simulink model "gap_generation_single_veh_state_machine"  (R2019a)
settings: Solver=VariableStepAuto  StartTime=0.0  StopTime=40  FixedStep=0.1  RelTol=1e-3
undefined symbols (not defined in the file): DiscIntNeverNeededParam
libraries: simulink x43, powerlib_meascontrol x5, autolibshared x5
(part 1 of 3)
settings Model: Creator=fvall  LastModifiedBy=fvall

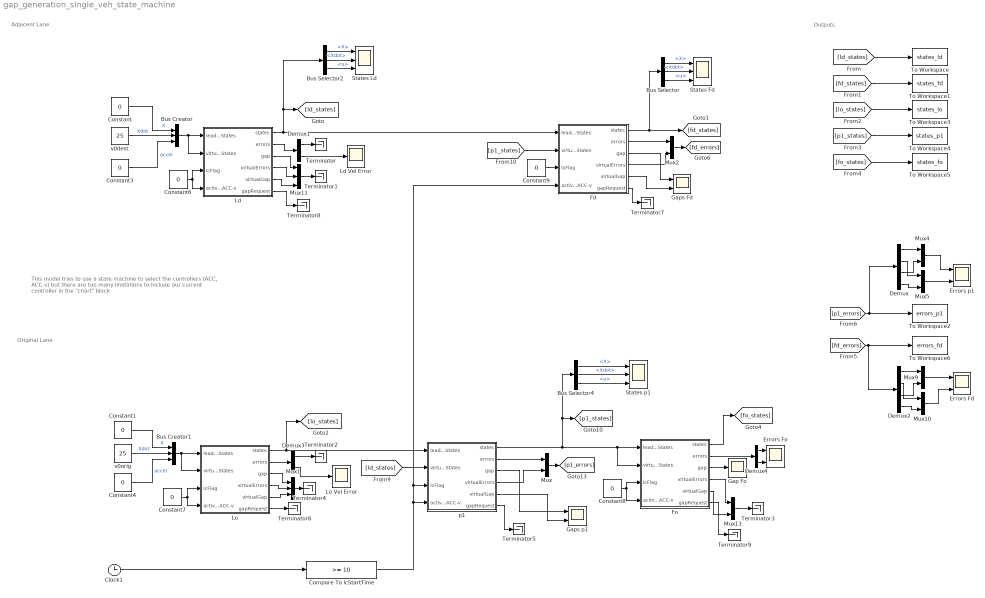
== system gap_generation_single_veh_state_machine ==
  note: Original Lane
  note: Adjacent Lane
  note: Outputs
  note: This model tries to use a state machine to select the controllers (ACC, ACC-v) but there are too many limitations to include our current controller in the "chart" block
  Bus Creator : BusCreator  Inputs=3
  Bus Creator1 : BusCreator  Inputs=3
  Bus Selector : BusSelector  OutputSignals=X,Xdot,u
  Bus Selector2 : BusSelector  OutputSignals=X,Xdot,u
  Bus Selector4 : BusSelector  OutputSignals=X,Xdot,u
  Clock1 : Clock
  Compare To lcStartTime : simulink/Logic and Bit Operations/Compare To Constant  relop=>=  const=10  OutDataTypeStr=boolean
  Constant{,1,3..4,6..9} (8 alike) : Constant  Value=0
  Demux : Demux
  Demux1 : Demux  Outputs=2
  Demux2 : Demux
  Demux3 : Demux  Outputs=2
  Demux4 : Demux  Outputs=2
  Errors Fd : Scope  NumInputPorts=2
  Errors Fo : Scope  NumInputPorts=2
  Errors p1 : Scope  NumInputPorts=2
  Fd : Subsystem  mask{m=2000, lf=2.5, lr=2.5, maxAcceleration=4, minAcceleration=-8, maxJerk=50, minJerk=-50, x0=20.2504, vx0=25, y0=3.6, h=0.63, d0=0.5004, minHeadwayError=-100, maxHeadwayError=3, velFilterGain=10, Kd=1.5652, Kp=2.2775, Ki=0.75, velKi=0.5, velKp=1.5, hFilterGain=0.5, vMin=18, l1=-2, maxComfAccel=2, minComfAccel=-2, maxComfJerk=10, minComfJerk=-10, hLc=2.215, d0Lc=0.5004}
      mask prompts: m "autoblks_shared:autoblkVehBody3DofLat:blkPrm_m"; lf "autoblks_shared:autoblkVehBody3DofLat:blkPrm_a"; lr "autoblks_shared:autoblkVehBody3DofLat:blkPrm_b"; maxAcceleration "Max Acceleration"; minAcceleration "Min Acceleration"; maxJerk "Max Jerk"; minJerk "Min Jerk"; x0 "autoblks_shared:autoblkVehBody3DofLat:blkPrm_X_o"; vx0 "autoblks_shared:autoblkVehBody3DofLat:blkPrm_xdot_o"; y0 "autoblks_shared:autoblkVehBody3DofLat:blkPrm_Y_o"; h "Time Headway"; d0 "Standstill Gap"; minHeadwayError "Min Headway Error"; maxHeadwayError "Max Headway Error"; velFilterGain "Velocity Filter Gain"; hFilterGain "Headway filter Gain"; vMin "Min Gap Gen Speed"; l1 "ACC-v Headway Error Threshold"; maxComfAccel "Max Comf Accel"; minComfAccel "Min Comf Accel"; maxComfJerk "Max Comf Jerk"; minComfJerk "Min Comf Jerk"; hLc "Time Headway LC"; d0Lc "Standstill Gap LC"
      mask TypeOptions m: Vehicle Body 3DOF Single Track/m
      mask TypeOptions lf: Vehicle Body 3DOF Single Track/a
      mask TypeOptions lr: Vehicle Body 3DOF Single Track/b
      mask TypeOptions x0: Vehicle Body 3DOF Single Track/X_o
      mask TypeOptions vx0: Vehicle Body 3DOF Single Track/xdot_o
      mask TypeOptions y0: Vehicle Body 3DOF Single Track/Y_o
      mask TypeOptions h: ACC/Headway error/h/Value
      mask TypeOptions d0: ACC/Headway error/d0/Value
      mask TypeOptions Kd: ACC/Kd/Gain
      mask TypeOptions Kp: ACC/Kp/Gain
      mask TypeOptions Ki: ACC/Ki/Gain
      mask TypeOptions velKi: ACC/velKi/Gain
      mask TypeOptions velKp: ACC/velKp/Gain
      mask TypeOptions hFilterGain: ACC/Headway error/hFilterGain/Gain
      mask TypeOptions vMin: ACC-v/vMin/Value
      mask TypeOptions l1:
      | ACC-v/Compare
      | To Constant/const
      mask TypeOptions hLc: ACC/Headway error/hLc/Value
      mask TypeOptions d0Lc: ACC/Headway error/d0Lc/Value
      mask DialogControl DescGroupVar Prompt: 3DOF Vehicle with ACC
      mask DialogControl DescTextVar Prompt: Vehicle with ACC. The vehicle model is Simulink's 3DOF single track vehicle body. The controller is a PID with constant headway including headway error saturation and filtered leader velocity.
      mask DialogControl VehParams Prompt: Vehicle Parameters
      mask DialogControl m Prompt: Vehicle mass, m [kg]:
      mask DialogControl lf Prompt: Longitudinal distance from center of mass to front axle, a [m]:
      mask DialogControl lr Prompt: Longitudinal distance from center of mass to rear axle, b [m]:
      mask DialogControl InitStates Prompt: Initial State
      mask DialogControl x0 Prompt: Initial inertial frame longitudinal position, X_o [m]:
      mask DialogControl vx0 Prompt: Initial longitudinal velocity, xdot_o [m/s]:
      mask DialogControl y0 Prompt: Initial inertial frame lateral displacement, Y_o [m]:
      mask DialogControl Container3 Prompt: Veh Following Parameters
      mask DialogControl VirtualFollParams Prompt: Virtual Veh Following Parameters
      mask DialogControl LCParams Prompt: Lane Change Params
  Fo : Subsystem  mask{m=2000, lf=2.5, lr=2.5, maxAcceleration=4, minAcceleration=-8, maxJerk=50, minJerk=-50, x0=0, vx0=25, y0=0, h=0.63, d0=0.5004, minHeadwayError=-100, maxHeadwayError=3, velFilterGain=10, Kd=1.5652, Kp=2.2775, Ki=0.75, velKi=0.5, velKp=1.5, hFilterGain=0.5, vMin=18, l1=-2, maxComfAccel=2, minComfAccel=-2, maxComfJerk=10, minComfJerk=-10, hLc=2.215, d0Lc=0.5004}
      mask prompts: m "autoblks_shared:autoblkVehBody3DofLat:blkPrm_m"; lf "autoblks_shared:autoblkVehBody3DofLat:blkPrm_a"; lr "autoblks_shared:autoblkVehBody3DofLat:blkPrm_b"; maxAcceleration "Max Acceleration"; minAcceleration "Min Acceleration"; maxJerk "Max Jerk"; minJerk "Min Jerk"; x0 "autoblks_shared:autoblkVehBody3DofLat:blkPrm_X_o"; vx0 "autoblks_shared:autoblkVehBody3DofLat:blkPrm_xdot_o"; y0 "autoblks_shared:autoblkVehBody3DofLat:blkPrm_Y_o"; h "Time Headway"; d0 "Standstill Gap"; minHeadwayError "Min Headway Error"; maxHeadwayError "Max Headway Error"; velFilterGain "Velocity Filter Gain"; hFilterGain "Headway filter Gain"; vMin "Min Gap Gen Speed"; l1 "ACC-v Headway Error Threshold"; maxComfAccel "Max Comf Accel"; minComfAccel "Min Comf Accel"; maxComfJerk "Max Comf Jerk"; minComfJerk "Min Comf Jerk"; hLc "Time Headway LC"; d0Lc "Standstill Gap LC"
      mask TypeOptions m: Vehicle Body 3DOF Single Track/m
      mask TypeOptions lf: Vehicle Body 3DOF Single Track/a
      mask TypeOptions lr: Vehicle Body 3DOF Single Track/b
      mask TypeOptions x0: Vehicle Body 3DOF Single Track/X_o
      mask TypeOptions vx0: Vehicle Body 3DOF Single Track/xdot_o
      mask TypeOptions y0: Vehicle Body 3DOF Single Track/Y_o
      mask TypeOptions h: ACC/Headway error/h/Value
      mask TypeOptions d0: ACC/Headway error/d0/Value
      mask TypeOptions Kd: ACC/Kd/Gain
      mask TypeOptions Kp: ACC/Kp/Gain
      mask TypeOptions Ki: ACC/Ki/Gain
      mask TypeOptions velKi: ACC/velKi/Gain
      mask TypeOptions velKp: ACC/velKp/Gain
      mask TypeOptions hFilterGain: ACC/Headway error/hFilterGain/Gain
      mask TypeOptions vMin: ACC-v/vMin/Value
      mask TypeOptions l1:
      | ACC-v/Compare
      | To Constant/const
      mask TypeOptions hLc: ACC/Headway error/hLc/Value
      mask TypeOptions d0Lc: ACC/Headway error/d0Lc/Value
      mask DialogControl DescGroupVar Prompt: 3DOF Vehicle with ACC
      mask DialogControl DescTextVar Prompt: Vehicle with ACC. The vehicle model is Simulink's 3DOF single track vehicle body. The controller is a PID with constant headway including headway error saturation and filtered leader velocity.
      mask DialogControl VehParams Prompt: Vehicle Parameters
      mask DialogControl m Prompt: Vehicle mass, m [kg]:
      mask DialogControl lf Prompt: Longitudinal distance from center of mass to front axle, a [m]:
      mask DialogControl lr Prompt: Longitudinal distance from center of mass to rear axle, b [m]:
      mask DialogControl InitStates Prompt: Initial State
      mask DialogControl x0 Prompt: Initial inertial frame longitudinal position, X_o [m]:
      mask DialogControl vx0 Prompt: Initial longitudinal velocity, xdot_o [m/s]:
      mask DialogControl y0 Prompt: Initial inertial frame lateral displacement, Y_o [m]:
      mask DialogControl Container3 Prompt: Veh Following Parameters
      mask DialogControl VirtualFollParams Prompt: Virtual Veh Following Parameters
      mask DialogControl LCParams Prompt: Lane Change Params
  Gap Fo : Scope
  Gaps Fd : Scope  NumInputPorts=2
  Gaps p1 : Scope  NumInputPorts=2
  Ld : Subsystem  mask{m=2000, lf=2.5, lr=2.5, maxAcceleration=4, minAcceleration=-8, maxJerk=50, minJerk=-50, x0=41.5008, vx0=25, y0=3.6, h=0.63, d0=0.5004, minHeadwayError=-100, maxHeadwayError=3, velFilterGain=10, Kd=1.5652, Kp=2.2775, Ki=0.75, velKi=0.5, velKp=1.5, hFilterGain=0.5, vMin=18, l1=-2, maxComfAccel=2, minComfAccel=-2, maxComfJerk=10, minComfJerk=-10, hLc=1.9025, d0Lc=0.5004}
      mask prompts: m "autoblks_shared:autoblkVehBody3DofLat:blkPrm_m"; lf "autoblks_shared:autoblkVehBody3DofLat:blkPrm_a"; lr "autoblks_shared:autoblkVehBody3DofLat:blkPrm_b"; maxAcceleration "Max Acceleration"; minAcceleration "Min Acceleration"; maxJerk "Max Jerk"; minJerk "Min Jerk"; x0 "autoblks_shared:autoblkVehBody3DofLat:blkPrm_X_o"; vx0 "autoblks_shared:autoblkVehBody3DofLat:blkPrm_xdot_o"; y0 "autoblks_shared:autoblkVehBody3DofLat:blkPrm_Y_o"; h "Time Headway"; d0 "Standstill Gap"; minHeadwayError "Min Headway Error"; maxHeadwayError "Max Headway Error"; velFilterGain "Velocity Filter Gain"; hFilterGain "Headway filter Gain"; vMin "Min Gap Gen Speed"; l1 "ACC-v Headway Error Threshold"; maxComfAccel "Max Comf Accel"; minComfAccel "Min Comf Accel"; maxComfJerk "Max Comf Jerk"; minComfJerk "Min Comf Jerk"; hLc "Time Headway LC"; d0Lc "Standstill Gap LC"
      mask TypeOptions m: Vehicle Body 3DOF Single Track/m
      mask TypeOptions lf: Vehicle Body 3DOF Single Track/a
      mask TypeOptions lr: Vehicle Body 3DOF Single Track/b
      mask TypeOptions x0: Vehicle Body 3DOF Single Track/X_o
      mask TypeOptions vx0: Vehicle Body 3DOF Single Track/xdot_o
      mask TypeOptions y0: Vehicle Body 3DOF Single Track/Y_o
      mask TypeOptions h: ACC/Headway error/h/Value
      mask TypeOptions d0: ACC/Headway error/d0/Value
      mask TypeOptions Kd: ACC/Kd/Gain
      mask TypeOptions Kp: ACC/Kp/Gain
      mask TypeOptions Ki: ACC/Ki/Gain
      mask TypeOptions velKi: ACC/velKi/Gain
      mask TypeOptions velKp: ACC/velKp/Gain
      mask TypeOptions hFilterGain: ACC/Headway error/hFilterGain/Gain
      mask TypeOptions vMin: ACC-v/vMin/Value
      mask TypeOptions l1:
      | ACC-v/Compare
      | To Constant/const
      mask TypeOptions hLc: ACC/Headway error/hLc/Value
      mask TypeOptions d0Lc: ACC/Headway error/d0Lc/Value
      mask DialogControl DescGroupVar Prompt: 3DOF Vehicle with ACC
      mask DialogControl DescTextVar Prompt: Vehicle with ACC. The vehicle model is Simulink's 3DOF single track vehicle body. The controller is a PID with constant headway including headway error saturation and filtered leader velocity.
      mask DialogControl VehParams Prompt: Vehicle Parameters
      mask DialogControl m Prompt: Vehicle mass, m [kg]:
      mask DialogControl lf Prompt: Longitudinal distance from center of mass to front axle, a [m]:
      mask DialogControl lr Prompt: Longitudinal distance from center of mass to rear axle, b [m]:
      mask DialogControl InitStates Prompt: Initial State
      mask DialogControl x0 Prompt: Initial inertial frame longitudinal position, X_o [m]:
      mask DialogControl vx0 Prompt: Initial longitudinal velocity, xdot_o [m/s]:
      mask DialogControl y0 Prompt: Initial inertial frame lateral displacement, Y_o [m]:
      mask DialogControl Container3 Prompt: Veh Following Parameters
      mask DialogControl VirtualFollParams Prompt: Virtual Veh Following Parameters
      mask DialogControl LCParams Prompt: Lane Change Params
  Ld Vel Error : Scope
  Lo : Subsystem  mask{m=2000, lf=2.5, lr=2.5, maxAcceleration=4, minAcceleration=-8, maxJerk=50, minJerk=-50, x0=42.5008, vx0=25, y0=0, h=0.63, d0=0.5004, minHeadwayError=-100, maxHeadwayError=3, velFilterGain=10, Kd=1.5652, Kp=2.2775, Ki=0.75, velKi=0.5, velKp=1.5, hFilterGain=0.5, vMin=18, l1=-2, maxComfAccel=2, minComfAccel=-2, maxComfJerk=10, minComfJerk=-10, hLc=1.9025, d0Lc=0.5004}
      mask prompts: m "autoblks_shared:autoblkVehBody3DofLat:blkPrm_m"; lf "autoblks_shared:autoblkVehBody3DofLat:blkPrm_a"; lr "autoblks_shared:autoblkVehBody3DofLat:blkPrm_b"; maxAcceleration "Max Acceleration"; minAcceleration "Min Acceleration"; maxJerk "Max Jerk"; minJerk "Min Jerk"; x0 "autoblks_shared:autoblkVehBody3DofLat:blkPrm_X_o"; vx0 "autoblks_shared:autoblkVehBody3DofLat:blkPrm_xdot_o"; y0 "autoblks_shared:autoblkVehBody3DofLat:blkPrm_Y_o"; h "Time Headway"; d0 "Standstill Gap"; minHeadwayError "Min Headway Error"; maxHeadwayError "Max Headway Error"; velFilterGain "Velocity Filter Gain"; hFilterGain "Headway filter Gain"; vMin "Min Gap Gen Speed"; l1 "ACC-v Headway Error Threshold"; maxComfAccel "Max Comf Accel"; minComfAccel "Min Comf Accel"; maxComfJerk "Max Comf Jerk"; minComfJerk "Min Comf Jerk"; hLc "Time Headway LC"; d0Lc "Standstill Gap LC"
      mask TypeOptions m: Vehicle Body 3DOF Single Track/m
      mask TypeOptions lf: Vehicle Body 3DOF Single Track/a
      mask TypeOptions lr: Vehicle Body 3DOF Single Track/b
      mask TypeOptions x0: Vehicle Body 3DOF Single Track/X_o
      mask TypeOptions vx0: Vehicle Body 3DOF Single Track/xdot_o
      mask TypeOptions y0: Vehicle Body 3DOF Single Track/Y_o
      mask TypeOptions h: ACC/Headway error/h/Value
      mask TypeOptions d0: ACC/Headway error/d0/Value
      mask TypeOptions Kd: ACC/Kd/Gain
      mask TypeOptions Kp: ACC/Kp/Gain
      mask TypeOptions Ki: ACC/Ki/Gain
      mask TypeOptions velKi: ACC/velKi/Gain
      mask TypeOptions velKp: ACC/velKp/Gain
      mask TypeOptions hFilterGain: ACC/Headway error/hFilterGain/Gain
      mask TypeOptions vMin: ACC-v/vMin/Value
      mask TypeOptions l1:
      | ACC-v/Compare
      | To Constant/const
      mask TypeOptions hLc: ACC/Headway error/hLc/Value
      mask TypeOptions d0Lc: ACC/Headway error/d0Lc/Value
      mask DialogControl DescGroupVar Prompt: 3DOF Vehicle with ACC
      mask DialogControl DescTextVar Prompt: Vehicle with ACC. The vehicle model is Simulink's 3DOF single track vehicle body. The controller is a PID with constant headway including headway error saturation and filtered leader velocity.
      mask DialogControl VehParams Prompt: Vehicle Parameters
      mask DialogControl m Prompt: Vehicle mass, m [kg]:
      mask DialogControl lf Prompt: Longitudinal distance from center of mass to front axle, a [m]:
      mask DialogControl lr Prompt: Longitudinal distance from center of mass to rear axle, b [m]:
      mask DialogControl InitStates Prompt: Initial State
      mask DialogControl x0 Prompt: Initial inertial frame longitudinal position, X_o [m]:
      mask DialogControl vx0 Prompt: Initial longitudinal velocity, xdot_o [m/s]:
      mask DialogControl y0 Prompt: Initial inertial frame lateral displacement, Y_o [m]:
      mask DialogControl Container3 Prompt: Veh Following Parameters
      mask DialogControl VirtualFollParams Prompt: Virtual Veh Following Parameters
      mask DialogControl LCParams Prompt: Lane Change Params
  Lo Vel Error : Scope
  Mux{,2,4..5,9..10,13} (7 alike) : Mux  Inputs=2
  Mux1 : Mux  Inputs=3
  Mux11 : Mux  Inputs=3
  States Fd : Scope  NumInputPorts=3
  States Ld : Scope  NumInputPorts=3
  States p1 : Scope  NumInputPorts=3
  Terminator{,1..9} (10 alike) : Terminator
  To Workspace : ToWorkspace  VariableName=states_ld  SampleTime=-1
  To Workspace1 : ToWorkspace  VariableName=states_fd  SampleTime=-1
  To Workspace2 : ToWorkspace  VariableName=errors_p1  SampleTime=-1
  To Workspace3 : ToWorkspace  VariableName=states_lo  SampleTime=-1
  To Workspace4 : ToWorkspace  VariableName=states_p1  SampleTime=-1
  To Workspace5 : ToWorkspace  VariableName=states_fo  SampleTime=-1
  To Workspace6 : ToWorkspace  VariableName=errors_fd  SampleTime=-1
  p1 : Subsystem  mask{m=2000, lf=2.5, lr=2.5, maxAcceleration=4, minAcceleration=-8, maxJerk=50, minJerk=-50, x0=21.2504, vx0=25, y0=0, h=0.63, d0=0.5004, minHeadwayError=-100, maxHeadwayError=3, velFilterGain=10, Kd=1.5652, Kp=2.2775, Ki=0.75, velKi=0.5, velKp=1.5, hFilterGain=0.5, vMin=18, l1=-2, maxComfAccel=2, minComfAccel=-2, maxComfJerk=10, minComfJerk=-10, hLc=2.215, d0Lc=0.5004}
      mask prompts: m "autoblks_shared:autoblkVehBody3DofLat:blkPrm_m"; lf "autoblks_shared:autoblkVehBody3DofLat:blkPrm_a"; lr "autoblks_shared:autoblkVehBody3DofLat:blkPrm_b"; maxAcceleration "Max Acceleration"; minAcceleration "Min Acceleration"; maxJerk "Max Jerk"; minJerk "Min Jerk"; x0 "autoblks_shared:autoblkVehBody3DofLat:blkPrm_X_o"; vx0 "autoblks_shared:autoblkVehBody3DofLat:blkPrm_xdot_o"; y0 "autoblks_shared:autoblkVehBody3DofLat:blkPrm_Y_o"; h "Time Headway"; d0 "Standstill Gap"; minHeadwayError "Min Headway Error"; maxHeadwayError "Max Headway Error"; velFilterGain "Velocity Filter Gain"; hFilterGain "Headway filter Gain"; vMin "Min Gap Gen Speed"; l1 "ACC-v Headway Error Threshold"; maxComfAccel "Max Comf Accel"; minComfAccel "Min Comf Accel"; maxComfJerk "Max Comf Jerk"; minComfJerk "Min Comf Jerk"; hLc "Time Headway LC"; d0Lc "Standstill Gap LC"
      mask TypeOptions m: Vehicle Body 3DOF Single Track/m
      mask TypeOptions lf: Vehicle Body 3DOF Single Track/a
      mask TypeOptions lr: Vehicle Body 3DOF Single Track/b
      mask TypeOptions x0: Vehicle Body 3DOF Single Track/X_o
      mask TypeOptions vx0: Vehicle Body 3DOF Single Track/xdot_o
      mask TypeOptions y0: Vehicle Body 3DOF Single Track/Y_o
      mask TypeOptions h: ACC/Headway error/h/Value
      mask TypeOptions d0: ACC/Headway error/d0/Value
      mask TypeOptions Kd: ACC/Kd/Gain
      mask TypeOptions Kp: ACC/Kp/Gain
      mask TypeOptions Ki: ACC/Ki/Gain
      mask TypeOptions velKi: ACC/velKi/Gain
      mask TypeOptions velKp: ACC/velKp/Gain
      mask TypeOptions hFilterGain: ACC/Headway error/hFilterGain/Gain
      mask TypeOptions vMin: ACC-v/vMin/Value
      mask TypeOptions l1:
      | ACC-v/Compare
      | To Constant/const
      mask TypeOptions hLc: ACC/Headway error/hLc/Value
      mask TypeOptions d0Lc: ACC/Headway error/d0Lc/Value
      mask DialogControl DescGroupVar Prompt: 3DOF Vehicle with ACC
      mask DialogControl DescTextVar Prompt: Vehicle with ACC. The vehicle model is Simulink's 3DOF single track vehicle body. The controller is a PID with constant headway including headway error saturation and filtered leader velocity.
      mask DialogControl VehParams Prompt: Vehicle Parameters
      mask DialogControl m Prompt: Vehicle mass, m [kg]:
      mask DialogControl lf Prompt: Longitudinal distance from center of mass to front axle, a [m]:
      mask DialogControl lr Prompt: Longitudinal distance from center of mass to rear axle, b [m]:
      mask DialogControl InitStates Prompt: Initial State
      mask DialogControl x0 Prompt: Initial inertial frame longitudinal position, X_o [m]:
      mask DialogControl vx0 Prompt: Initial longitudinal velocity, xdot_o [m/s]:
      mask DialogControl y0 Prompt: Initial inertial frame lateral displacement, Y_o [m]:
      mask DialogControl Container3 Prompt: Veh Following Parameters
      mask DialogControl VirtualFollParams Prompt: Virtual Veh Following Parameters
      mask DialogControl LCParams Prompt: Lane Change Params
  v0dest : Constant  Value=25
  v0orig : Constant  Value=25
  wires:
  Clock1/1 -> Compare To lcStartTime/1
  Lo/1(states) -> p1/1(leaderStates), [lo_states]
  Bus Selector4/3 -> States p1/3  "<u>"
  Bus Selector4/2 -> States p1/2  "<Xdot>"
  Bus Selector4/1 -> States p1/1  "<X>"
  p1/2(errors) -> Mux/1
  Ld/2(errors) -> Demux1/1
  Bus Selector2/3 -> States Ld/3  "<u>"
  Fd/6(gapRequest) -> Terminator7/1
  Fd/4(virtualErrors) -> Mux2/2
  Fd/5(virtualGap) -> Gaps Fd/2
  Fd/1(states) -> Bus Selector/1, [fd_states]
  Ld/3(gap) -> Mux11/1
  Fd/3(gap) -> Gaps Fd/1
  Mux11/1 -> Terminator1/1
  Fd/2(errors) -> Mux2/1
  Demux1/2 -> Ld Vel Error/1
  Bus Selector2/2 -> States Ld/2  "<Xdot>"
  Bus Selector2/1 -> States Ld/1  "<X>"
  Ld/6(gapRequest) -> Terminator8/1
  Bus Selector/1 -> States Fd/1  "<X>"
  [p1_states] -> Fd/2(virtualLeaderStates)
  Constant9/1 -> Fd/3(lcFlag)
  Ld/5(virtualGap) -> Mux11/3
  Bus Selector/3 -> States Fd/3  "<u>"
  Constant6/1 -> Ld/4(activate ACC-v), Ld/3(lcFlag)
  Ld/4(virtualErrors) -> Mux11/2
  Bus Selector/2 -> States Fd/2  "<Xdot>"
  Ld/1(states) -> Fd/1(leaderStates), Bus Selector2/1, [ld_states]
  v0dest/1 -> Bus Creator/2  "Xdot"
  Constant3/1 -> Bus Creator/3  "accel"
  Mux2/1 -> [fd_errors]
  Constant/1 -> Bus Creator/1  "X"
  Demux1/1 -> Terminator/1
  Bus Creator/1 -> Ld/1(leaderStates), Ld/2(virtualLeaderStates)
  Lo/2(errors) -> Demux3/1
  Demux3/1 -> Terminator2/1
  Bus Creator1/1 -> Lo/1(leaderStates), Lo/2(virtualLeaderStates)
  Constant7/1 -> Lo/3(lcFlag), Lo/4(activate ACC-v)
  v0orig/1 -> Bus Creator1/2  "Xdot"
  Constant4/1 -> Bus Creator1/3  "accel"
  Constant1/1 -> Bus Creator1/1  "X"
  Demux3/2 -> Lo Vel Error/1
  Mux13/1 -> Terminator3/1
  Fo/2(errors) -> Demux4/1
  Fo/4(virtualErrors) -> Mux13/1
  Fo/3(gap) -> Gap Fo/1
  Demux4/2 -> Errors Fo/2
  Constant8/1 -> Fo/4(activate ACC-v), Fo/3(lcFlag)
  Demux4/1 -> Errors Fo/1
  Fo/1(states) -> [fo_states]
  p1/1(states) -> Fo/2(virtualLeaderStates), Fo/1(leaderStates), Bus Selector4/1, [p1_states]
  Fo/5(virtualGap) -> Mux13/2
  [ld_states] -> p1/2(virtualLeaderStates)
  Compare To lcStartTime/1 -> Fd/4(activate ACC-v), p1/3(lcFlag), p1/4(activate ACC-v)
  p1/3(gap) -> Gaps p1/1
  [fd_states] -> To Workspace1/1
  [lo_states] -> To Workspace3/1
  Mux10/1 -> Errors Fd/2
  Mux4/1 -> Errors p1/1
  Demux/2 -> Mux5/1
  Mux9/1 -> Errors Fd/1
  Demux/3 -> Mux4/2
  Demux/1 -> Mux4/1
  Mux5/1 -> Errors p1/2
  Demux2/2 -> Mux10/1
  Demux2/3 -> Mux9/2
  [p1_errors] -> To Workspace2/1, Demux/1
  [fd_errors] -> Demux2/1, To Workspace6/1
  [p1_states] -> To Workspace4/1
  Demux2/4 -> Mux10/2
  [ld_states] -> To Workspace/1
  Demux/4 -> Mux5/2
  [fo_states] -> To Workspace5/1
  Demux2/1 -> Mux9/1
  Mux/1 -> [p1_errors]
  p1/4(virtualErrors) -> Mux/2
  p1/5(virtualGap) -> Gaps p1/2
  p1/6(gapRequest) -> Terminator5/1
  Lo/3(gap) -> Mux1/1
  Lo/4(virtualErrors) -> Mux1/2
  Lo/5(virtualGap) -> Mux1/3
  Mux1/1 -> Terminator4/1
  Lo/6(gapRequest) -> Terminator6/1
  Fo/6(gapRequest) -> Terminator9/1

== system gap_generation_single_veh_state_machine/Fd ==
  leaderStates : Inport
  virtualLeaderStates : Inport  Port=2
  lcFlag : Inport  Port=3
  activate ACC-v : Inport  Port=4
  ACC : Subsystem
  ACC-v : Subsystem
  AND : Logic  Inputs=3  IconShape=distinctive  AllPortsSameDT=off  OutDataTypeStr=boolean
  Abs : Abs
  Abs1 : Abs  ZeroCross=off
  Bus Creator : BusCreator  Inputs=4
  Bus Selector : BusSelector  OutputSignals=InertFrm.RearAxl.Disp.X,InertFrm.RearAxl.Disp.Y,InertFrm.RearAxl.Vel.Xdot
  Compare To Constant : simulink/Logic and Bit Operations/Compare To Constant  relop=<=  const=0.5  OutDataTypeStr=boolean
  Compare To Constant1 : simulink/Logic and Bit Operations/Compare To Constant  relop=<=  const=0.5  OutDataTypeStr=boolean
  Constant : Constant  Value=0
  Constant1 : Constant  Value=maxAcceleration+1
  Gain : Gain  Gain=m/2
  Min : MinMax  Inputs=2
  Mux1 : Mux  Inputs=6
  On Delay : powerlib_meascontrol/Logic/On Delay  DelayType=On delay  delay=1  ic=0  Ts=0
      settings: SourceProductName=Simscape Electrical
  Scope : Scope  NumInputPorts=2
  Scope1 : Scope  NumInputPorts=3
  Signal Specification : SignalSpecification  Dimensions=1
  Switch : Switch  Criteria=u2 > Threshold
  Terminator : Terminator
  Transport Delay : TransportDelay
  Triggered Subsystem : Subsystem  TreatAsAtomicUnit=on
  Vehicle Body 3DOF Single Track : autolibshared/Vehicle Body 3DOF Single Track  trackMode=Single (bicycle)  inputMode=External longitudinal forces  frontSteerMode=on  rearSteerMode=off  windMode=off  muMode=off  extFMode=off  extMMode=off  extXo=off  extpsio=off  extxdoto=off  extro=off  extYo=off  extTamb=off  extydoto=off  aMode=2  NF=2  NR=2  m=m  a=lf  b=lr  h=0.35  X_o=x0  xdot_o=vx0  CalphaMode=off  sigmaMode=on  d=0  w=[1.4,1.4]  Cy_f=12e3  Cy_r=11e3  sigma_f=.1  sigma_r=.1  alpha_f_brk=[-.1 .1]  Cy_f_data=[-9e3 9e3]  alpha_r_brk=[-.1 .1]  Cy_r_data=[-9e3 9e3]  Y_o=y0  ydot_o=0  Izz=4000  psi_o=0  r_o=0  Af=2  Cd=.3  Cl=.1  Cpm=.1  beta_w=[0:0.01:0.3]  Cs=[0:0.03:0.9]  Cym=[0:0.01:0.3]  Pabs=101325  Tair=273  g=9.81  mu=1  xdot_tol=.01  Fznom=5000  Fxtire_sat=7e4  Fytire_sat=7e4  longOff=0  latOff=0  vertOff=0  wrapAng=off
      settings: SourceProductName=Powertrain Blockset  SourceProductBaseCode=PW
  states : Outport
  errors : Outport  Port=2
  gap : Outport  Port=3
  virtualErrors : Outport  Port=4
  virtualGap : Outport  Port=5
  gapRequest : Outport  Port=6
  wires:
  Abs1/1 -> Compare To Constant1/1
  Abs/1 -> Compare To Constant/1
  Transport Delay/1 -> Abs/1
  Compare To Constant/1 -> AND/2
  Triggered Subsystem/1(Out1) -> Scope/2, gapRequest/1
  On Delay/1 -> Triggered Subsystem/1(In1), AND/3
  Compare To Constant1/1 -> AND/1, Scope/1
  AND/1 -> Triggered Subsystem/Trigger
  Constant1/1 -> Switch/3
  activate ACC-v/1 -> Switch/2, ACC-v/3(activate)
  Signal Specification/1 -> Gain/1, Bus Creator/4, Abs1/1, Transport Delay/1
  Bus Selector/2 -> Bus Creator/2  "<Y>"
  ACC-v/3(gap) -> virtualGap/1
  ACC-v/2(errors) -> virtualErrors/1
  ACC-v/1(u) -> Switch/1
  Switch/1 -> Min/2, Scope1/2  "acc-v"
  lcFlag/1 -> ACC/3(lcFlag), On Delay/1, ACC-v/4(lcFlag)
  ACC/2(errors) -> errors/1
  virtualLeaderStates/1 -> ACC-v/2(leaderStates)
  leaderStates/1 -> ACC/2(leaderStates)
  Bus Creator/1 -> states/1, ACC-v/1(currentStates), ACC/1(currentStates)
  ACC/3(gap) -> gap/1
  Mux1/1 -> Terminator/1
  Vehicle Body 3DOF Single Track/7 -> Mux1/6
  Vehicle Body 3DOF Single Track/6 -> Mux1/5
  Vehicle Body 3DOF Single Track/5 -> Mux1/4
  Vehicle Body 3DOF Single Track/2 -> Mux1/1
  Vehicle Body 3DOF Single Track/3 -> Mux1/2
  Vehicle Body 3DOF Single Track/4 -> Mux1/3
  Vehicle Body 3DOF Single Track/1 -> Bus Selector/1
  Constant/1 -> Vehicle Body 3DOF Single Track/1
  Gain/1 -> Vehicle Body 3DOF Single Track/2, Vehicle Body 3DOF Single Track/3
  ACC/1(u) -> Min/1, Scope1/1  "acc"
  Min/1 -> Signal Specification/1, Scope1/3  "u"
  Bus Selector/1 -> Bus Creator/1  "<X>"
  Bus Selector/3 -> Bus Creator/3  "<Xdot>"

== system gap_generation_single_veh_state_machine/Fo ==
  leaderStates : Inport
  virtualLeaderStates : Inport  Port=2
  lcFlag : Inport  Port=3
  activate ACC-v : Inport  Port=4
  ACC : Subsystem
  ACC-v : Subsystem
  AND : Logic  Inputs=3  IconShape=distinctive  AllPortsSameDT=off  OutDataTypeStr=boolean
  Abs : Abs
  Abs1 : Abs  ZeroCross=off
  Bus Creator : BusCreator  Inputs=4
  Bus Selector : BusSelector  OutputSignals=InertFrm.RearAxl.Disp.X,InertFrm.RearAxl.Disp.Y,InertFrm.RearAxl.Vel.Xdot
  Compare To Constant : simulink/Logic and Bit Operations/Compare To Constant  relop=<=  const=0.5  OutDataTypeStr=boolean
  Compare To Constant1 : simulink/Logic and Bit Operations/Compare To Constant  relop=<=  const=0.5  OutDataTypeStr=boolean
  Constant : Constant  Value=0
  Constant1 : Constant  Value=maxAcceleration+1
  Gain : Gain  Gain=m/2
  Min : MinMax  Inputs=2
  Mux1 : Mux  Inputs=6
  On Delay : powerlib_meascontrol/Logic/On Delay  DelayType=On delay  delay=1  ic=0  Ts=0
      settings: SourceProductName=Simscape Electrical
  Scope : Scope  NumInputPorts=2
  Scope1 : Scope  NumInputPorts=3
  Signal Specification : SignalSpecification  Dimensions=1
  Switch : Switch  Criteria=u2 > Threshold
  Terminator : Terminator
  Transport Delay : TransportDelay
  Triggered Subsystem : Subsystem  TreatAsAtomicUnit=on
  Vehicle Body 3DOF Single Track : autolibshared/Vehicle Body 3DOF Single Track  trackMode=Single (bicycle)  inputMode=External longitudinal forces  frontSteerMode=on  rearSteerMode=off  windMode=off  muMode=off  extFMode=off  extMMode=off  extXo=off  extpsio=off  extxdoto=off  extro=off  extYo=off  extTamb=off  extydoto=off  aMode=2  NF=2  NR=2  m=m  a=lf  b=lr  h=0.35  X_o=x0  xdot_o=vx0  CalphaMode=off  sigmaMode=on  d=0  w=[1.4,1.4]  Cy_f=12e3  Cy_r=11e3  sigma_f=.1  sigma_r=.1  alpha_f_brk=[-.1 .1]  Cy_f_data=[-9e3 9e3]  alpha_r_brk=[-.1 .1]  Cy_r_data=[-9e3 9e3]  Y_o=y0  ydot_o=0  Izz=4000  psi_o=0  r_o=0  Af=2  Cd=.3  Cl=.1  Cpm=.1  beta_w=[0:0.01:0.3]  Cs=[0:0.03:0.9]  Cym=[0:0.01:0.3]  Pabs=101325  Tair=273  g=9.81  mu=1  xdot_tol=.01  Fznom=5000  Fxtire_sat=7e4  Fytire_sat=7e4  longOff=0  latOff=0  vertOff=0  wrapAng=off
      settings: SourceProductName=Powertrain Blockset  SourceProductBaseCode=PW
  states : Outport
  errors : Outport  Port=2
  gap : Outport  Port=3
  virtualErrors : Outport  Port=4
  virtualGap : Outport  Port=5
  gapRequest : Outport  Port=6
  wires:
  Abs1/1 -> Compare To Constant1/1
  Abs/1 -> Compare To Constant/1
  Transport Delay/1 -> Abs/1
  Compare To Constant/1 -> AND/2
  Triggered Subsystem/1(Out1) -> Scope/2, gapRequest/1
  On Delay/1 -> Triggered Subsystem/1(In1), AND/3
  Compare To Constant1/1 -> AND/1, Scope/1
  AND/1 -> Triggered Subsystem/Trigger
  Constant1/1 -> Switch/3
  activate ACC-v/1 -> Switch/2, ACC-v/3(activate)
  Signal Specification/1 -> Gain/1, Bus Creator/4, Abs1/1, Transport Delay/1
  Bus Selector/2 -> Bus Creator/2  "<Y>"
  ACC-v/3(gap) -> virtualGap/1
  ACC-v/2(errors) -> virtualErrors/1
  ACC-v/1(u) -> Switch/1
  Switch/1 -> Min/2, Scope1/2  "acc-v"
  lcFlag/1 -> ACC/3(lcFlag), On Delay/1, ACC-v/4(lcFlag)
  ACC/2(errors) -> errors/1
  virtualLeaderStates/1 -> ACC-v/2(leaderStates)
  leaderStates/1 -> ACC/2(leaderStates)
  Bus Creator/1 -> states/1, ACC-v/1(currentStates), ACC/1(currentStates)
  ACC/3(gap) -> gap/1
  Mux1/1 -> Terminator/1
  Vehicle Body 3DOF Single Track/7 -> Mux1/6
  Vehicle Body 3DOF Single Track/6 -> Mux1/5
  Vehicle Body 3DOF Single Track/5 -> Mux1/4
  Vehicle Body 3DOF Single Track/2 -> Mux1/1
  Vehicle Body 3DOF Single Track/3 -> Mux1/2
  Vehicle Body 3DOF Single Track/4 -> Mux1/3
  Vehicle Body 3DOF Single Track/1 -> Bus Selector/1
  Constant/1 -> Vehicle Body 3DOF Single Track/1
  Gain/1 -> Vehicle Body 3DOF Single Track/2, Vehicle Body 3DOF Single Track/3
  ACC/1(u) -> Min/1, Scope1/1  "acc"
  Min/1 -> Signal Specification/1, Scope1/3  "u"
  Bus Selector/1 -> Bus Creator/1  "<X>"
  Bus Selector/3 -> Bus Creator/3  "<Xdot>"

== system gap_generation_single_veh_state_machine/Ld ==
  leaderStates : Inport
  virtualLeaderStates : Inport  Port=2
  lcFlag : Inport  Port=3
  activate ACC-v : Inport  Port=4
  ACC : Subsystem
  ACC-v : Subsystem
  AND : Logic  Inputs=3  IconShape=distinctive  AllPortsSameDT=off  OutDataTypeStr=boolean
  Abs : Abs
  Abs1 : Abs  ZeroCross=off
  Bus Creator : BusCreator  Inputs=4  OutDataTypeStr=Bus: vehStates
  Bus Selector : BusSelector  OutputSignals=InertFrm.RearAxl.Disp.X,InertFrm.RearAxl.Disp.Y,InertFrm.RearAxl.Vel.Xdot
  Compare To Constant : simulink/Logic and Bit Operations/Compare To Constant  relop=<=  const=0.5  OutDataTypeStr=boolean
  Compare To Constant1 : simulink/Logic and Bit Operations/Compare To Constant  relop=<=  const=0.5  OutDataTypeStr=boolean
  Constant : Constant  Value=0
  Constant1 : Constant  Value=maxAcceleration+1
  Gain : Gain  Gain=m/2
  Min : MinMax  Inputs=2
  Mux1 : Mux  Inputs=6
  On Delay : powerlib_meascontrol/Logic/On Delay  DelayType=On delay  delay=1  ic=0  Ts=0
      settings: SourceProductName=Simscape Electrical
  Scope : Scope  NumInputPorts=2
  Scope1 : Scope  NumInputPorts=3
  Signal Specification : SignalSpecification  Dimensions=1
  Switch : Switch  Criteria=u2 > Threshold
  Terminator : Terminator
  Transport Delay : TransportDelay
  Triggered Subsystem : Subsystem  TreatAsAtomicUnit=on
  Vehicle Body 3DOF Single Track : autolibshared/Vehicle Body 3DOF Single Track  trackMode=Single (bicycle)  inputMode=External longitudinal forces  frontSteerMode=on  rearSteerMode=off  windMode=off  muMode=off  extFMode=off  extMMode=off  extXo=off  extpsio=off  extxdoto=off  extro=off  extYo=off  extTamb=off  extydoto=off  aMode=2  NF=2  NR=2  m=m  a=lf  b=lr  h=0.35  X_o=x0  xdot_o=vx0  CalphaMode=off  sigmaMode=on  d=0  w=[1.4,1.4]  Cy_f=12e3  Cy_r=11e3  sigma_f=.1  sigma_r=.1  alpha_f_brk=[-.1 .1]  Cy_f_data=[-9e3 9e3]  alpha_r_brk=[-.1 .1]  Cy_r_data=[-9e3 9e3]  Y_o=y0  ydot_o=0  Izz=4000  psi_o=0  r_o=0  Af=2  Cd=.3  Cl=.1  Cpm=.1  beta_w=[0:0.01:0.3]  Cs=[0:0.03:0.9]  Cym=[0:0.01:0.3]  Pabs=101325  Tair=273  g=9.81  mu=1  xdot_tol=.01  Fznom=5000  Fxtire_sat=7e4  Fytire_sat=7e4  longOff=0  latOff=0  vertOff=0  wrapAng=off
      settings: SourceProductName=Powertrain Blockset  SourceProductBaseCode=PW
  states : Outport
  errors : Outport  Port=2
  gap : Outport  Port=3
  virtualErrors : Outport  Port=4
  virtualGap : Outport  Port=5
  gapRequest : Outport  Port=6
  wires:
  Bus Selector/3 -> Bus Creator/3  "<Xdot>"
  Bus Selector/1 -> Bus Creator/1  "<X>"
  Min/1 -> Scope1/3, Signal Specification/1  "u"
  ACC/1(u) -> Scope1/1, Min/1  "acc"
  Gain/1 -> Vehicle Body 3DOF Single Track/3, Vehicle Body 3DOF Single Track/2
  Constant/1 -> Vehicle Body 3DOF Single Track/1
  Vehicle Body 3DOF Single Track/1 -> Bus Selector/1
  Vehicle Body 3DOF Single Track/4 -> Mux1/3
  Vehicle Body 3DOF Single Track/3 -> Mux1/2
  Vehicle Body 3DOF Single Track/2 -> Mux1/1
  Vehicle Body 3DOF Single Track/5 -> Mux1/4
  Vehicle Body 3DOF Single Track/6 -> Mux1/5
  Vehicle Body 3DOF Single Track/7 -> Mux1/6
  Mux1/1 -> Terminator/1
  ACC/3(gap) -> gap/1
  Bus Creator/1 -> ACC/1(currentStates), ACC-v/1(currentStates), states/1
  leaderStates/1 -> ACC/2(leaderStates)
  virtualLeaderStates/1 -> ACC-v/2(leaderStates)
  ACC/2(errors) -> errors/1
  lcFlag/1 -> ACC-v/4(lcFlag), On Delay/1, ACC/3(lcFlag)
  Switch/1 -> Scope1/2, Min/2  "acc-v"
  ACC-v/1(u) -> Switch/1
  ACC-v/2(errors) -> virtualErrors/1
  ACC-v/3(gap) -> virtualGap/1
  Bus Selector/2 -> Bus Creator/2  "<Y>"
  Signal Specification/1 -> Transport Delay/1, Abs1/1, Bus Creator/4, Gain/1
  activate ACC-v/1 -> ACC-v/3(activate), Switch/2
  Constant1/1 -> Switch/3
  AND/1 -> Triggered Subsystem/Trigger
  Compare To Constant1/1 -> Scope/1, AND/1
  On Delay/1 -> AND/3, Triggered Subsystem/1(In1)
  Triggered Subsystem/1(Out1) -> gapRequest/1, Scope/2
  Compare To Constant/1 -> AND/2
  Transport Delay/1 -> Abs/1
  Abs/1 -> Compare To Constant/1
  Abs1/1 -> Compare To Constant1/1

== system gap_generation_single_veh_state_machine/Lo ==
  leaderStates : Inport
  virtualLeaderStates : Inport  Port=2
  lcFlag : Inport  Port=3
  activate ACC-v : Inport  Port=4
  ACC : Subsystem
  ACC-v : Subsystem
  AND : Logic  Inputs=3  IconShape=distinctive  AllPortsSameDT=off  OutDataTypeStr=boolean
  Abs : Abs
  Abs1 : Abs  ZeroCross=off
  Bus Creator : BusCreator  Inputs=4  OutDataTypeStr=Bus: vehStates
  Bus Selector : BusSelector  OutputSignals=InertFrm.RearAxl.Disp.X,InertFrm.RearAxl.Disp.Y,InertFrm.RearAxl.Vel.Xdot
  Compare To Constant : simulink/Logic and Bit Operations/Compare To Constant  relop=<=  const=0.5  OutDataTypeStr=boolean
  Compare To Constant1 : simulink/Logic and Bit Operations/Compare To Constant  relop=<=  const=0.5  OutDataTypeStr=boolean
  Constant : Constant  Value=0
  Constant1 : Constant  Value=maxAcceleration+1
  Gain : Gain  Gain=m/2
  Min : MinMax  Inputs=2
  Mux1 : Mux  Inputs=6
  On Delay : powerlib_meascontrol/Logic/On Delay  DelayType=On delay  delay=1  ic=0  Ts=0
      settings: SourceProductName=Simscape Electrical
  Scope : Scope  NumInputPorts=2
  Scope1 : Scope  NumInputPorts=3
  Signal Specification : SignalSpecification  Dimensions=1
  Switch : Switch  Criteria=u2 > Threshold
  Terminator : Terminator
  Transport Delay : TransportDelay
  Triggered Subsystem : Subsystem  TreatAsAtomicUnit=on
  Vehicle Body 3DOF Single Track : autolibshared/Vehicle Body 3DOF Single Track  trackMode=Single (bicycle)  inputMode=External longitudinal forces  frontSteerMode=on  rearSteerMode=off  windMode=off  muMode=off  extFMode=off  extMMode=off  extXo=off  extpsio=off  extxdoto=off  extro=off  extYo=off  extTamb=off  extydoto=off  aMode=2  NF=2  NR=2  m=m  a=lf  b=lr  h=0.35  X_o=x0  xdot_o=vx0  CalphaMode=off  sigmaMode=on  d=0  w=[1.4,1.4]  Cy_f=12e3  Cy_r=11e3  sigma_f=.1  sigma_r=.1  alpha_f_brk=[-.1 .1]  Cy_f_data=[-9e3 9e3]  alpha_r_brk=[-.1 .1]  Cy_r_data=[-9e3 9e3]  Y_o=y0  ydot_o=0  Izz=4000  psi_o=0  r_o=0  Af=2  Cd=.3  Cl=.1  Cpm=.1  beta_w=[0:0.01:0.3]  Cs=[0:0.03:0.9]  Cym=[0:0.01:0.3]  Pabs=101325  Tair=273  g=9.81  mu=1  xdot_tol=.01  Fznom=5000  Fxtire_sat=7e4  Fytire_sat=7e4  longOff=0  latOff=0  vertOff=0  wrapAng=off
      settings: SourceProductName=Powertrain Blockset  SourceProductBaseCode=PW
  states : Outport
  errors : Outport  Port=2
  gap : Outport  Port=3
  virtualErrors : Outport  Port=4
  virtualGap : Outport  Port=5
  gapRequest : Outport  Port=6
  wires:
  Abs1/1 -> Compare To Constant1/1
  Abs/1 -> Compare To Constant/1
  Transport Delay/1 -> Abs/1
  Compare To Constant/1 -> AND/2
  Triggered Subsystem/1(Out1) -> Scope/2, gapRequest/1
  On Delay/1 -> Triggered Subsystem/1(In1), AND/3
  Compare To Constant1/1 -> AND/1, Scope/1
  AND/1 -> Triggered Subsystem/Trigger
  Constant1/1 -> Switch/3
  activate ACC-v/1 -> Switch/2, ACC-v/3(activate)
  Signal Specification/1 -> Gain/1, Bus Creator/4, Abs1/1, Transport Delay/1
  Bus Selector/2 -> Bus Creator/2  "<Y>"
  ACC-v/3(gap) -> virtualGap/1
  ACC-v/2(errors) -> virtualErrors/1
  ACC-v/1(u) -> Switch/1
  Switch/1 -> Min/2, Scope1/2  "acc-v"
  lcFlag/1 -> ACC/3(lcFlag), On Delay/1, ACC-v/4(lcFlag)
  ACC/2(errors) -> errors/1
  virtualLeaderStates/1 -> ACC-v/2(leaderStates)
  leaderStates/1 -> ACC/2(leaderStates)
  Bus Creator/1 -> states/1, ACC-v/1(currentStates), ACC/1(currentStates)
  ACC/3(gap) -> gap/1
  Mux1/1 -> Terminator/1
  Vehicle Body 3DOF Single Track/7 -> Mux1/6
  Vehicle Body 3DOF Single Track/6 -> Mux1/5
  Vehicle Body 3DOF Single Track/5 -> Mux1/4
  Vehicle Body 3DOF Single Track/2 -> Mux1/1
  Vehicle Body 3DOF Single Track/3 -> Mux1/2
  Vehicle Body 3DOF Single Track/4 -> Mux1/3
  Vehicle Body 3DOF Single Track/1 -> Bus Selector/1
  Constant/1 -> Vehicle Body 3DOF Single Track/1
  Gain/1 -> Vehicle Body 3DOF Single Track/2, Vehicle Body 3DOF Single Track/3
  ACC/1(u) -> Min/1, Scope1/1  "acc"
  Min/1 -> Signal Specification/1, Scope1/3  "u"
  Bus Selector/1 -> Bus Creator/1  "<X>"
  Bus Selector/3 -> Bus Creator/3  "<Xdot>"

== system gap_generation_single_veh_state_machine/p1 ==
  leaderStates : Inport
  virtualLeaderStates : Inport  Port=2
  lcFlag : Inport  Port=3
  activate ACC-v : Inport  Port=4
  ACC : Subsystem
  AND : Logic  Inputs=3  IconShape=distinctive  AllPortsSameDT=off  OutDataTypeStr=boolean
  Abs : Abs
  Abs1 : Abs  ZeroCross=off
  Bus Creator : BusCreator  Inputs=4  OutDataTypeStr=Bus: vehStates
  Bus Selector : BusSelector  OutputSignals=InertFrm.RearAxl.Disp.X,InertFrm.RearAxl.Disp.Y,InertFrm.RearAxl.Vel.Xdot
  Chart : Stateflow chart  BlockKeywords=__PRM__SERIALIZED__DATA__:Stateflow Chart,Stateflow Diagram  TreatAsAtomicUnit=on
  Compare To Constant : simulink/Logic and Bit Operations/Compare To Constant  relop=<=  const=0.5  OutDataTypeStr=boolean
  Compare To Constant1 : simulink/Logic and Bit Operations/Compare To Constant  relop=<=  const=0.5  OutDataTypeStr=boolean
  Constant : Constant  Value=0
  Demux : Demux  Outputs=2
  Enabled Subsystem : Subsystem  TreatAsAtomicUnit=on
  Gain : Gain  Gain=m/2
  Min : MinMax  Inputs=2
  Mux1 : Mux  Inputs=6
  NOT : Logic  Operator=NOT  IconShape=distinctive  AllPortsSameDT=off  OutDataTypeStr=boolean
  On Delay : powerlib_meascontrol/Logic/On Delay  DelayType=On delay  delay=1  ic=0  Ts=0
      settings: SourceProductName=Simscape Electrical
  Rate Limiter1 : RateLimiter  RisingSlewLimit=10  FallingSlewLimit=-10  SampleTimeMode=inherited
  Scope : Scope  NumInputPorts=2
  Scope1 : Scope  NumInputPorts=3
  Scope2 : Scope  NumInputPorts=2
  Signal Specification : SignalSpecification  Dimensions=1
  Switch : Switch  Criteria=u2 > Threshold
  Terminator : Terminator
  Transport Delay : TransportDelay
  Triggered Subsystem : Subsystem  TreatAsAtomicUnit=on
  Vehicle Body 3DOF Single Track : autolibshared/Vehicle Body 3DOF Single Track  trackMode=Single (bicycle)  inputMode=External longitudinal forces  frontSteerMode=on  rearSteerMode=off  windMode=off  muMode=off  extFMode=off  extMMode=off  extXo=off  extpsio=off  extxdoto=off  extro=off  extYo=off  extTamb=off  extydoto=off  aMode=2  NF=2  NR=2  m=m  a=lf  b=lr  h=0.35  X_o=x0  xdot_o=vx0  CalphaMode=off  sigmaMode=on  d=0  w=[1.4,1.4]  Cy_f=12e3  Cy_r=11e3  sigma_f=.1  sigma_r=.1  alpha_f_brk=[-.1 .1]  Cy_f_data=[-9e3 9e3]  alpha_r_brk=[-.1 .1]  Cy_r_data=[-9e3 9e3]  Y_o=y0  ydot_o=0  Izz=4000  psi_o=0  r_o=0  Af=2  Cd=.3  Cl=.1  Cpm=.1  beta_w=[0:0.01:0.3]  Cs=[0:0.03:0.9]  Cym=[0:0.01:0.3]  Pabs=101325  Tair=273  g=9.81  mu=1  xdot_tol=.01  Fznom=5000  Fxtire_sat=7e4  Fytire_sat=7e4  longOff=0  latOff=0  vertOff=0  wrapAng=off
      settings: SourceProductName=Powertrain Blockset  SourceProductBaseCode=PW
  eh stateflow : Scope  NumInputPorts=2
  ev stateflow : Scope  NumInputPorts=2
  gap stateflow : Scope
  states : Outport
  errors : Outport  Port=2
  gap : Outport  Port=3
  virtualErrors : Outport  Port=4
  virtualGap : Outport  Port=5
  gapRequest : Outport  Port=6
  wires:
  Bus Selector/3 -> Bus Creator/3  "<Xdot>"
  Bus Selector/1 -> Bus Creator/1  "<X>"
  Gain/1 -> Vehicle Body 3DOF Single Track/3, Vehicle Body 3DOF Single Track/2
  Constant/1 -> Vehicle Body 3DOF Single Track/1
  Vehicle Body 3DOF Single Track/1 -> Bus Selector/1
  Vehicle Body 3DOF Single Track/4 -> Mux1/3
  Vehicle Body 3DOF Single Track/3 -> Mux1/2
  Vehicle Body 3DOF Single Track/2 -> Mux1/1
  Vehicle Body 3DOF Single Track/5 -> Mux1/4
  Vehicle Body 3DOF Single Track/6 -> Mux1/5
  Vehicle Body 3DOF Single Track/7 -> Mux1/6
  Mux1/1 -> Terminator/1
  ACC/3(gap) -> gap/1
  Bus Creator/1 -> ACC/1(currentStates), Chart/1(currentStates), Enabled Subsystem/1(currentStates), states/1
  leaderStates/1 -> Chart/2(leaderStates), ACC/2(leaderStates)
  virtualLeaderStates/1 -> Chart/5(virtualLeaderStates), Enabled Subsystem/2(leaderStates)
  ACC/2(errors) -> Demux/1, errors/1
  lcFlag/1 -> ACC/3(lcFlag), Chart/3(lcFlag), Enabled Subsystem/4(lcFlag), On Delay/1
  Enabled Subsystem/2(errors) -> virtualErrors/1
  Enabled Subsystem/3(gap) -> virtualGap/1
  Bus Selector/2 -> Bus Creator/2  "<Y>"
  activate ACC-v/1 -> Chart/4(virtualFollowing), NOT/1, Enabled Subsystem/Enable, Enabled Subsystem/3(activate)
  AND/1 -> Triggered Subsystem/Trigger
  Compare To Constant1/1 -> Scope/1, AND/1
  On Delay/1 -> AND/3, Triggered Subsystem/1(In1)
  Triggered Subsystem/1(Out1) -> gapRequest/1, Scope/2
  Compare To Constant/1 -> AND/2
  Transport Delay/1 -> Abs/1
  Abs/1 -> Compare To Constant/1
  Abs1/1 -> Compare To Constant1/1
  Min/1 -> Signal Specification/1, Scope1/3  "u"
  Enabled Subsystem/1(u) -> Rate Limiter1/1
  ACC/1(u) -> Switch/1, Scope1/1, Min/1  "acc"
  NOT/1 -> Switch/2
  Signal Specification/1 -> Switch/3
  Rate Limiter1/1 -> Scope1/2, Min/2  "acc-v"
  Chart/4(gap) -> gap stateflow/1
  Chart/2(eh) -> eh stateflow/1
  Chart/3(ev) -> ev stateflow/1
  Demux/1 -> eh stateflow/2
  Demux/2 -> ev stateflow/2
  Chart/1(u) -> Gain/1, Bus Creator/4, Abs1/1, Transport Delay/1, Scope2/2  "u"
  Switch/1 -> Scope2/1  "u"

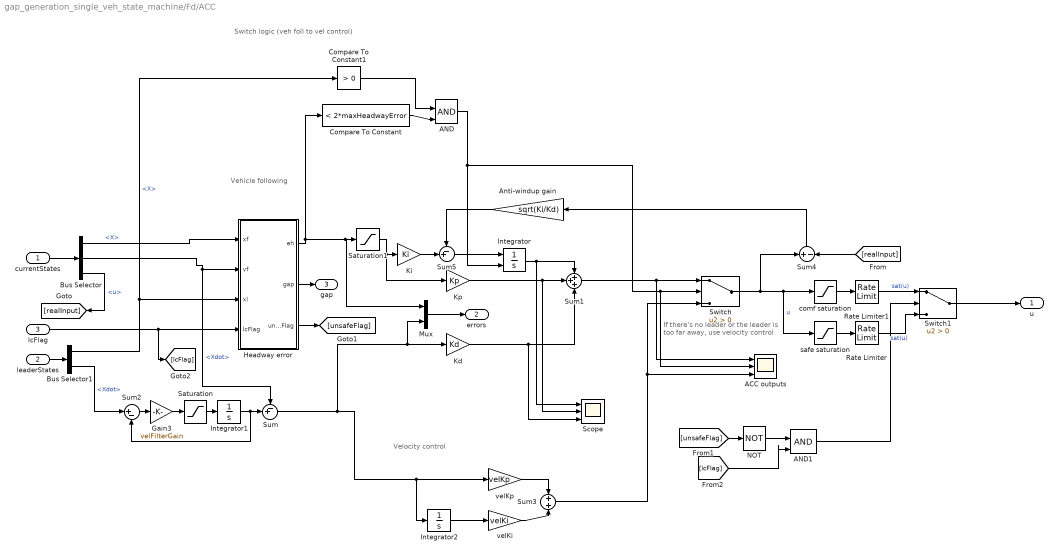
== system gap_generation_single_veh_state_machine/Fd/ACC ==
  note: If there's no leader or the leader
      | is too far away, use velocity control
  note: Velocity control
  note: Switch logic (veh foll to vel control)
  note: Vehicle following
  currentStates : Inport
  leaderStates : Inport  Port=2
  lcFlag : Inport  Port=3
  ACC outputs : Scope  NumInputPorts=3
  AND : Logic  IconShape=distinctive  AllPortsSameDT=off  OutDataTypeStr=boolean
  AND1 : Logic  IconShape=distinctive  AllPortsSameDT=off  OutDataTypeStr=boolean
  Anti-windup gain : Gain  Gain=sqrt(Ki/Kd)
  Bus Selector : BusSelector  OutputSignals=X,Xdot,u
  Bus Selector1 : BusSelector  OutputSignals=X,Xdot
  Compare To Constant : simulink/Logic and Bit Operations/Compare To Constant  relop=<  const=2*maxHeadwayError  OutDataTypeStr=boolean
  Compare To Constant1 : simulink/Logic and Bit Operations/Compare To Constant  relop=>  const=0  OutDataTypeStr=boolean
  Gain3 : Gain  Gain=velFilterGain
  Headway error : Subsystem
  Integrator : Integrator  ExternalReset=either
  Integrator1 : Integrator  InitialCondition=vx0
  Integrator2 : Integrator
  Kd : Gain  Gain=Kd
  Ki : Gain  Gain=Ki
  Kp : Gain  Gain=Kp
  Mux : Mux  Inputs=2
  NOT : Logic  Operator=NOT  IconShape=distinctive  AllPortsSameDT=off  OutDataTypeStr=boolean
  Rate Limiter : RateLimiter  RisingSlewLimit=maxComfJerk  FallingSlewLimit=minComfJerk  SampleTimeMode=inherited
  Rate Limiter1 : RateLimiter  RisingSlewLimit=10  FallingSlewLimit=-10  SampleTimeMode=inherited
  Saturation : Saturate  UpperLimit=maxAcceleration  LowerLimit=minAcceleration
  Saturation1 : Saturate  UpperLimit=maxHeadwayError  LowerLimit=minHeadwayError
  Scope : Scope  NumInputPorts=3
  Sum : Sum  Inputs=-+|
  Sum1 : Sum  Inputs=+++
  Sum2 : Sum  Inputs=|+-
  Sum3 : Sum
  Sum4 : Sum  Inputs=+-
  Sum5 : Sum  Inputs=-+|
  Switch : Switch  Criteria=u2 > Threshold
  Switch1 : Switch  Criteria=u2 > Threshold
  comf saturation : Saturate  UpperLimit=2  LowerLimit=-2
  safe saturation : Saturate  UpperLimit=maxComfAccel  LowerLimit=minComfAccel
  velKi : Gain  Gain=velKi
  velKp : Gain  Gain=velKp
  u : Outport
  errors : Outport  Port=2
  gap : Outport  Port=3
  wires:
  Rate Limiter1/1 -> Switch1/1  "sat(u)"
  Switch1/1 -> u/1
  Rate Limiter/1 -> Switch1/3  "sat(u)"
  safe saturation/1 -> Rate Limiter/1
  AND1/1 -> Switch1/2
  comf saturation/1 -> Rate Limiter1/1
  [lcFlag] -> AND1/2
  NOT/1 -> AND1/1
  [unsafeFlag] -> NOT/1
  Headway error/3(unsafeFlag) -> [unsafeFlag]
  [realInput] -> Sum4/2
  Bus Selector/3 -> [realInput]  "<u>"
  Bus Selector1/1 -> Headway error/3(xl), Compare To Constant1/1  "<X>"
  leaderStates/1 -> Bus Selector1/1
  Bus Selector/1 -> Headway error/1(xf)  "<X>"
  currentStates/1 -> Bus Selector/1
  lcFlag/1 -> Headway error/4(lcFlag), [lcFlag]
  Compare To Constant1/1 -> AND/1
  Compare To Constant/1 -> AND/2
  AND/1 -> ACC outputs/2, Switch/2, Integrator/2
  Anti-windup gain/1 -> Sum5/1
  Integrator/1 -> Scope/1, Sum1/1
  Ki/1 -> Sum5/2
  velKp/1 -> Sum3/1
  Sum5/1 -> Integrator/1
  Sum4/1 -> Anti-windup gain/1
  Mux/1 -> errors/1
  Sum/1 -> Integrator2/1, velKp/1, Kd/1, Mux/2
  Sum3/1 -> Switch/3, ACC outputs/3
  Sum1/1 -> ACC outputs/1, Switch/1
  Switch/1 -> comf saturation/1, safe saturation/1, Sum4/1  "u"
  velKi/1 -> Sum3/2
  Integrator2/1 -> velKi/1
  Headway error/2("gap ") -> gap/1
  Saturation1/1 -> Ki/1, Kp/1
  Sum2/1 -> Gain3/1
  Bus Selector1/2 -> Sum2/1  "<Xdot>"
  Integrator1/1 -> Sum/2, Sum2/2
  Saturation/1 -> Integrator1/1
  Gain3/1 -> Saturation/1
  Kp/1 -> Sum1/2, Scope/2
  Kd/1 -> Sum1/3, Scope/3
  Bus Selector/2 -> Sum/1, Headway error/2(vf)  "<Xdot>"
  Headway error/1(eh) -> Compare To Constant/1, Mux/1, Saturation1/1
